simulink model "sampleModel1816"  (R2023a)
settings: Solver=VariableStepAuto  StartTime=0.0  StopTime=10.0  RelTol=1e-3
libraries: hdlsllib x7, simulink x2
settings Model: Creator=user1  LastModifiedBy=user1

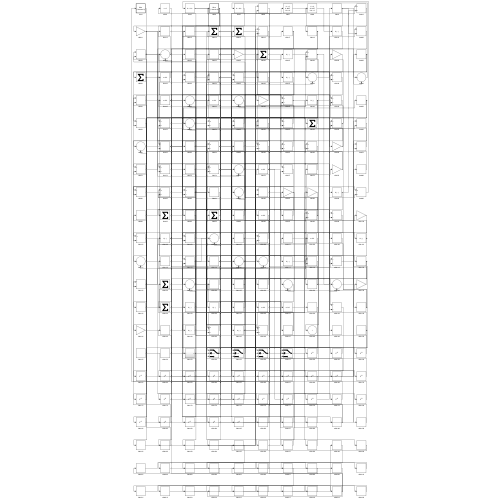
[thumbnail: Simulink's stored preview of the top-level diagram]
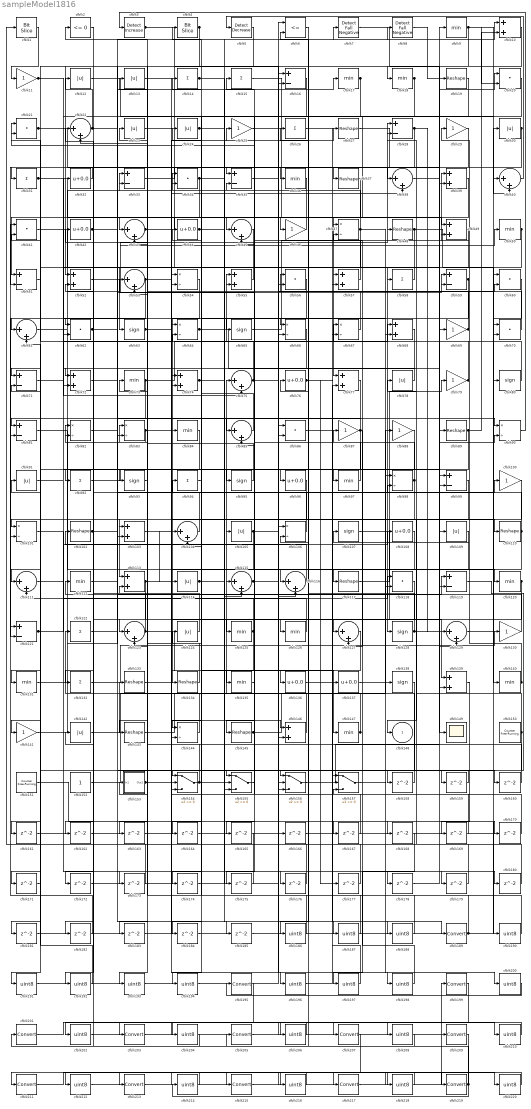
== system sampleModel1816 ==
  cfblk1 : hdlsllib/Logic and Bit Operations/Bit Slice  lidx=7  ridx=0
  cfblk{10,39,49,52,55,57,68,72,74,77,103,113,139,146} (14 alike) : Sum
  cfblk{11,25,29,46,69,79,87..88,100,130,141} (11 alike) : Gain
  cfblk{47,54,64,66..67,82..83,90,98,101,106,144} (12 alike) : Product  Inputs=*/  RndMeth=Zero  SaturateOnIntegerOverflow=on
  cfblk{19,27,37,48,89,102,110,117,133..134,143,145} (12 alike) : Reshape
  cfblk{22,38,40,43,45,53,61,75,85,104,111,115..116,123,127,129} (16 alike) : Sum  Inputs=|++
  cfblk{12..13,23..24,30,78,91,105,109,114,124,142} (12 alike) : Abs  SaturateOnIntegerOverflow=off
  cfblk{63,65,80,93,95,107,128,138} (8 alike) : Signum
  cfblk{32,42,44,76,96,108,136..137} (8 alike) : Bias  Bias=0.0  SaturateOnIntegerOverflow=off
  cfblk{9,17..18,36,50,73,84,97,112,120,125..126,131,135,140,147} (16 alike) : MinMax
  cfblk{20..21,34,41,56,60,62,70,86,118} (10 alike) : DotProduct  OutDataTypeStr=Inherit: Inherit via internal rule
  cfblk{16,28,33,35,51,59,71,81,99,119,121} (11 alike) : Sum  Inputs=+-
  cfblk{14..15,26,31,58,92,94,122,132} (9 alike) : Sum  Inputs=+
  cfblk149 : Scope
  cfblk150 : hdlsllib/Sources/Counter Free-Running  NumBits=16  tsamp=-1
  cfblk151 : hdlsllib/Sources/Counter Free-Running  NumBits=16  tsamp=-1
  cfblk152 : Constant  SampleTime=-1
  cfblk153 : Subsystem
      settings: LibrarySourceBlock=|
      | hdlsllib/Ports &
      | Subsystems/Subsystem
  cfblk{154..157} (4 alike) : Switch  SaturateOnIntegerOverflow=off  InputSameDT=off
  cfblk{158..185} (28 alike) : Delay  SampleTime=1
  cfblk{186..188,190..194,196..198,200,202,204,206,208,210,212,214,216,218,220} (22 alike) : DataTypeConversion  OutDataTypeStr=uint8  SaturateOnIntegerOverflow=off  RndMeth=Floor
  cfblk{189,195,199,201,203,205,207,209,211,213,215,217,219} (13 alike) : DataTypeConversion  SaturateOnIntegerOverflow=off  RndMeth=Floor
  cfblk2 : hdlsllib/Logic and Bit Operations/Compare To Zero  relop=<=  OutDataTypeStr=boolean
  cfblk3 : simulink/Logic and Bit Operations/Detect Increase  vinit=0.0  OutDataTypeStr=boolean
      settings: LibrarySourceBlock=|
      | hdlsllib/Logic and Bit
      | Operations/Detect
      | Increase
  cfblk4 : hdlsllib/Logic and Bit Operations/Bit Slice  lidx=7  ridx=0
  cfblk5 : simulink/Logic and Bit Operations/Detect Decrease  vinit=0.0  OutDataTypeStr=boolean
      settings: LibrarySourceBlock=|
      | hdlsllib/Logic and Bit
      | Operations/Detect
      | Decrease
  cfblk6 : RelationalOperator  Operator=<=  OutDataTypeStr=boolean  InputSameDT=off
  cfblk7 : hdlsllib/Logic and Bit Operations/Detect Fall Negative  vinit=0  OutDataTypeStr=boolean
  cfblk8 : hdlsllib/Logic and Bit Operations/Detect Fall Negative  vinit=0  OutDataTypeStr=boolean
  cfblk148 : Outport  VectorParamsAs1DForOutWhenUnconnected=off
  wires:
  cfblk113/1 -> cfblk123/1, cfblk104/1, cfblk118/2
  cfblk54/1 -> cfblk134/1
  cfblk105/1 -> cfblk114/1, cfblk68/1
  cfblk17/1 -> cfblk62/2, cfblk182/1
  cfblk8/1 -> cfblk19/1
  cfblk92/1 -> cfblk96/1
  cfblk34/1 -> cfblk51/1, cfblk156/3, cfblk188/1
  cfblk81/1 -> cfblk120/1
  cfblk144/1 -> cfblk73/1
  cfblk131/1 -> cfblk33/1
  cfblk10/1 -> cfblk52/1
  cfblk130/1 -> cfblk112/1
  cfblk76/1 -> cfblk99/2, cfblk177/1
  cfblk18/1 -> cfblk46/1, cfblk163/1
  cfblk32/1 -> cfblk31/1
  cfblk65/1 -> cfblk39/1
  cfblk132/1 -> cfblk130/1
  cfblk2/1 -> cfblk92/1
  cfblk98/1 -> cfblk113/1, cfblk21/2, cfblk53/1
  cfblk146/1 -> cfblk122/1
  cfblk55/1 -> cfblk63/1
  cfblk97/1 -> cfblk87/1
  cfblk143/1 -> cfblk75/1
  cfblk41/1 -> cfblk128/1
  cfblk19/1 -> cfblk125/1
  cfblk91/1 -> cfblk95/1
  cfblk33/1 -> cfblk35/1
  cfblk30/1 -> cfblk37/1, cfblk56/2
  cfblk123/1 -> cfblk147/1, cfblk146/2, cfblk82/1
  cfblk133/1 -> cfblk25/1
  cfblk95/1 -> cfblk23/1
  cfblk142/1 -> cfblk133/1
  cfblk77/1 -> cfblk121/2
  cfblk25/1 -> cfblk77/1
  cfblk111/1 -> cfblk105/1
  cfblk117/1 -> cfblk79/1
  cfblk110/1 -> cfblk59/1, cfblk144/1
  cfblk46/1 -> cfblk45/1
  cfblk119/1 -> cfblk154/1
  cfblk150/1 -> cfblk78/1, cfblk154/3
  cfblk96/1 -> cfblk141/1
  cfblk84/1 -> cfblk93/1
  cfblk79/1 -> cfblk55/1, cfblk41/2
  cfblk9/1 -> cfblk18/1, cfblk20/2, cfblk40/2
  cfblk48/1 -> cfblk140/1, cfblk71/1, cfblk81/1, cfblk62/1
  cfblk141/1 -> cfblk119/1
  cfblk88/1 -> cfblk103/1
  cfblk4/1 -> cfblk43/1, cfblk83/2, cfblk101/1
  cfblk107/1 -> cfblk139/1
  cfblk37/1 -> cfblk132/1
  cfblk5/1 -> cfblk103/2
  cfblk28/1 -> cfblk116/1, cfblk129/1
  cfblk134/1 -> cfblk2/1
  cfblk155/1 -> cfblk115/1
  cfblk62/1 -> cfblk59/2, cfblk65/1, cfblk176/1
  cfblk114/1 -> cfblk100/1, cfblk10/1
  cfblk61/1 -> cfblk28/1
  cfblk116/1 -> cfblk102/1
  cfblk43/1 -> cfblk47/1, cfblk49/1
  cfblk72/1 -> cfblk90/1
  cfblk108/1 -> cfblk135/1
  cfblk115/1 -> cfblk60/2, cfblk159/1
  cfblk64/1 -> cfblk155/2, cfblk109/1
  cfblk40/1 -> cfblk5/1
  cfblk73/1 -> cfblk67/1, cfblk101/2
  cfblk140/1 -> cfblk94/1, cfblk107/1
  cfblk21/1 -> cfblk38/1, cfblk58/1
  cfblk87/1 -> cfblk127/2, cfblk85/1, cfblk191/1
  cfblk118/1 -> cfblk126/1
  cfblk100/1 -> cfblk148/1
  cfblk78/1 -> cfblk72/1
  cfblk50/1 -> cfblk131/1, cfblk143/1
  cfblk14/1 -> cfblk167/1, cfblk168/1
  cfblk104/1 -> cfblk22/1
  cfblk99/1 -> cfblk136/1
  cfblk44/1 -> cfblk84/1, cfblk104/2, cfblk156/1
  cfblk124/1 -> cfblk83/1
  cfblk3/1 -> cfblk139/2, cfblk106/1
  cfblk137/1 -> cfblk138/1
  cfblk128/1 -> cfblk76/1, cfblk90/2
  cfblk152/1 -> cfblk98/1
  cfblk1/1 -> cfblk11/1
  cfblk68/1 -> cfblk72/2
  cfblk135/1 -> cfblk15/1
  cfblk56/1 -> cfblk66/1
  cfblk47/1 -> cfblk33/2, cfblk85/2, cfblk180/1
  cfblk57/1 -> cfblk35/2
  cfblk102/1 -> cfblk98/2, cfblk187/1
  cfblk69/1 -> cfblk42/1, cfblk49/2
  cfblk147/1 -> cfblk56/1, cfblk4/1
  cfblk129/1 -> cfblk80/1
  cfblk153/1(Out1) -> cfblk108/1, cfblk183/1
  cfblk109/1 -> cfblk119/2
  cfblk94/1 -> cfblk14/1
  cfblk70/1 -> cfblk22/2
  cfblk12/1 -> cfblk40/1
  cfblk27/1 -> cfblk89/1
  cfblk53/1 -> cfblk38/2, cfblk81/2
  cfblk154/1 -> cfblk48/1, cfblk53/2
  cfblk63/1 -> cfblk54/2, cfblk110/1
  cfblk86/1 -> cfblk189/1
  cfblk80/1 -> cfblk34/1
  cfblk38/1 -> cfblk20/1
  cfblk49/1 -> cfblk111/1
  cfblk121/1 -> cfblk64/2, cfblk118/1
  cfblk120/1 -> cfblk144/2, cfblk172/1
  cfblk7/1 -> cfblk69/1
  cfblk106/1 -> cfblk45/2
  cfblk145/1 -> cfblk88/1, cfblk198/1
  cfblk58/1 -> cfblk57/1
  cfblk156/1 -> cfblk9/1
  cfblk15/1 -> cfblk149/1
  cfblk52/1 -> cfblk50/1
  cfblk36/1 -> cfblk74/2
  cfblk90/1 -> cfblk3/1
  cfblk67/1 -> cfblk26/1
  cfblk60/1 -> cfblk70/2
  cfblk85/1 -> cfblk24/1
  cfblk89/1 -> cfblk10/2, cfblk184/1
  cfblk82/1 -> cfblk7/1
  cfblk125/1 -> cfblk111/2, cfblk194/1
  cfblk31/1 -> cfblk67/2, cfblk171/1
  cfblk22/1 -> cfblk36/1, cfblk12/1
  cfblk24/1 -> cfblk8/1, cfblk39/2
  cfblk29/1 -> cfblk51/2
  cfblk74/1 -> cfblk129/2, cfblk27/1, cfblk160/1
  cfblk66/1 -> cfblk145/1
  cfblk13/1 -> cfblk57/2
  cfblk71/1 -> cfblk32/1
  cfblk83/1 -> cfblk127/1, cfblk43/2, cfblk137/1, cfblk146/1, cfblk82/2
  cfblk75/1 -> cfblk21/1, cfblk117/1
  cfblk126/1 -> cfblk44/1
  cfblk11/1 -> cfblk61/1, cfblk75/2, cfblk68/2
  cfblk122/1 -> cfblk17/1
  cfblk42/1 -> cfblk97/1, cfblk156/2
  cfblk59/1 -> cfblk29/1, cfblk174/1
  cfblk103/1 -> cfblk158/1
  cfblk158/1 -> cfblk113/2
  cfblk159/1 -> cfblk155/1
  cfblk160/1 -> cfblk123/2
  cfblk51/1 -> cfblk161/1
  cfblk161/1 -> cfblk34/2
  cfblk45/1 -> cfblk162/1
  cfblk162/1 -> cfblk70/1
  cfblk20/1 -> cfblk164/1
  cfblk164/1 -> cfblk115/2
  cfblk127/1 -> cfblk165/1
  cfblk165/1 -> cfblk1/1
  cfblk35/1 -> cfblk166/1
  cfblk166/1 -> cfblk60/1
  cfblk167/1 -> cfblk55/2
  cfblk139/1 -> cfblk169/1
  cfblk169/1 -> cfblk54/1
  cfblk26/1 -> cfblk170/1
  cfblk170/1 -> cfblk47/2
  cfblk171/1 -> cfblk71/2
  cfblk172/1 -> cfblk116/2
  cfblk101/1 -> cfblk173/1
  cfblk173/1 -> cfblk52/2
  cfblk174/1 -> cfblk155/3
  cfblk39/1 -> cfblk175/1
  cfblk175/1 -> cfblk64/1
  cfblk176/1 -> cfblk154/2
  cfblk177/1 -> cfblk41/1
  cfblk136/1 -> cfblk178/1
  cfblk178/1 -> cfblk99/1
  cfblk23/1 -> cfblk179/1
  cfblk179/1 -> cfblk28/2
  cfblk180/1 -> cfblk61/2
  cfblk138/1 -> cfblk181/1
  cfblk181/1 -> cfblk74/1
  cfblk182/1 -> cfblk121/1
  cfblk183/1 -> cfblk77/2
  cfblk184/1 -> cfblk66/2
  cfblk112/1 -> cfblk185/1
  cfblk185/1 -> cfblk30/1
  cfblk6/1 -> cfblk186/1
  cfblk186/1 -> cfblk124/1
  cfblk187/1 -> cfblk6/1
  cfblk188/1 -> cfblk6/2
  cfblk189/1 -> cfblk153/1(In1), cfblk13/1
  cfblk151/1 -> cfblk190/1
  cfblk190/1 -> cfblk86/1
  cfblk191/1 -> cfblk86/2
  cfblk16/1 -> cfblk192/1
  cfblk192/1 -> cfblk91/1
  cfblk93/1 -> cfblk193/1
  cfblk193/1 -> cfblk16/1
  cfblk194/1 -> cfblk16/2
  cfblk163/1 -> cfblk196/1
  cfblk196/1 -> cfblk157/1
  cfblk168/1 -> cfblk197/1
  cfblk197/1 -> cfblk157/2
  cfblk198/1 -> cfblk157/3
  cfblk157/1 -> cfblk200/1
  cfblk200/1 -> cfblk195/1
  cfblk195/1 -> cfblk202/1
  cfblk202/1 -> cfblk199/1
  cfblk199/1 -> cfblk204/1
  cfblk204/1 -> cfblk201/1
  cfblk201/1 -> cfblk206/1
  cfblk206/1 -> cfblk203/1
  cfblk203/1 -> cfblk208/1
  cfblk208/1 -> cfblk205/1
  cfblk205/1 -> cfblk210/1
  cfblk210/1 -> cfblk207/1
  cfblk207/1 -> cfblk212/1
  cfblk212/1 -> cfblk209/1
  cfblk209/1 -> cfblk214/1
  cfblk214/1 -> cfblk211/1
  cfblk211/1 -> cfblk216/1
  cfblk216/1 -> cfblk213/1
  cfblk217/1 -> cfblk219/1
  cfblk213/1 -> cfblk218/1
  cfblk218/1 -> cfblk215/1
  cfblk219/1 -> cfblk142/1, cfblk106/2
  cfblk215/1 -> cfblk220/1
  cfblk220/1 -> cfblk217/1

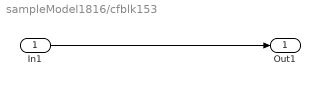
== system sampleModel1816/cfblk153 ==
  In1 : Inport
  Out1 : Outport
  wires:
  In1/1 -> Out1/1
